simulink model "AM6"  (R2020b)
settings: Solver=VariableStepDiscrete  StartTime=0.0  StopTime=2  MaxStep=1e-6  RelTol=1e-3
undefined symbols (not defined in the file or in its folder): offset
settings Model: Creator=seojoon  LastModifiedBy=seojoon

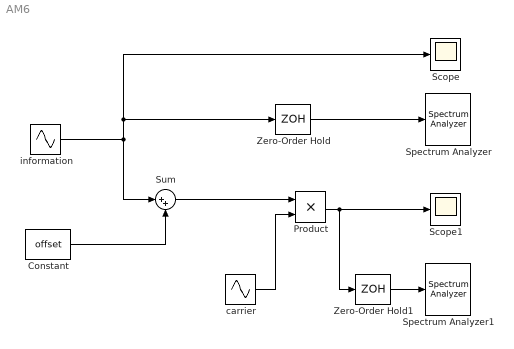
== system AM6 ==
  Constant : Constant  Value=offset  VectorParams1D=off
  Product : Product
  Scope : Scope
  Scope1 : Scope
  Spectrum Analyzer : SpectrumAnalyzer
  Spectrum Analyzer1 : SpectrumAnalyzer
  Sum : Sum  Inputs=|++
  Zero-Order Hold : ZeroOrderHold  SampleTime=1/2000
  Zero-Order Hold1 : ZeroOrderHold  SampleTime=1/2000
  carrier : Sin  Frequency=2*pi*100  Phase=pi/2  SampleTime=0
  information : Sin  Amplitude=2  Frequency=2*pi*5  SampleTime=0
  wires:
  information/1 -> Sum/1, Scope/1, Zero-Order Hold/1
  Constant/1 -> Sum/2
  Sum/1 -> Product/1
  carrier/1 -> Product/2
  Product/1 -> Zero-Order Hold1/1, Scope1/1
  Zero-Order Hold/1 -> Spectrum Analyzer/1
  Zero-Order Hold1/1 -> Spectrum Analyzer1/1
